simulink model "RCAMSimulation"  (R2025b)
settings: Solver=VariableStepAuto  StartTime=0.0  StopTime=TF  RelTol=1e-3
values from neighbouring files (symbols this model uses):
  u1max = 25*pi/180    (= 0.436332312999)    [Initialize_RCAM.m]
  u1min = -25*pi/180    (= -0.436332312999)    [Initialize_RCAM.m]
  u2max = 10*pi/180    (= 0.174532925199)    [Initialize_RCAM.m]
  u2min = -25*pi/180    (= -0.436332312999)    [Initialize_RCAM.m]
  u3max = 30*pi/180    (= 0.523598775598)    [Initialize_RCAM.m]
  u3min = -30*pi/180    (= -0.523598775598)    [Initialize_RCAM.m]
  u4max = 10*pi/180    (= 0.174532925199)    [Initialize_RCAM.m]
  u4min = 0    [Initialize_RCAM.m]
  u5max = 10*pi/180    (= 0.174532925199)    [Initialize_RCAM.m]
  u5min = 0.5*pi/180    (= 0.00872664625997)    [Initialize_RCAM.m]
  x0 = [85;0;0;0;0;0;0;0.1;0]    [Initialize_RCAM.m]
undefined symbols (not defined in the file or in its folder): RCAM_model
libraries: aerolibsim3d x2, sim3dlib x1
settings Model: Creator=andyf  LastModifiedBy=andyf

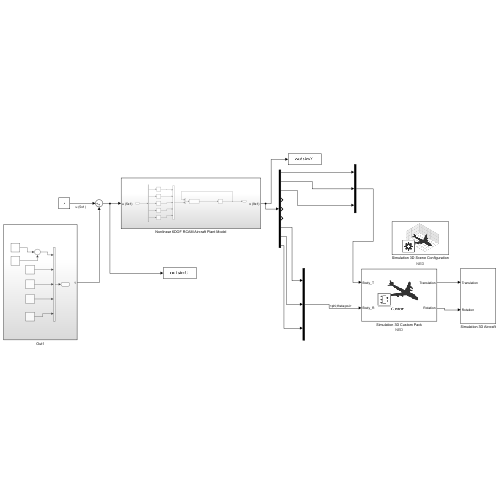
[thumbnail: Simulink's stored preview of the top-level diagram]
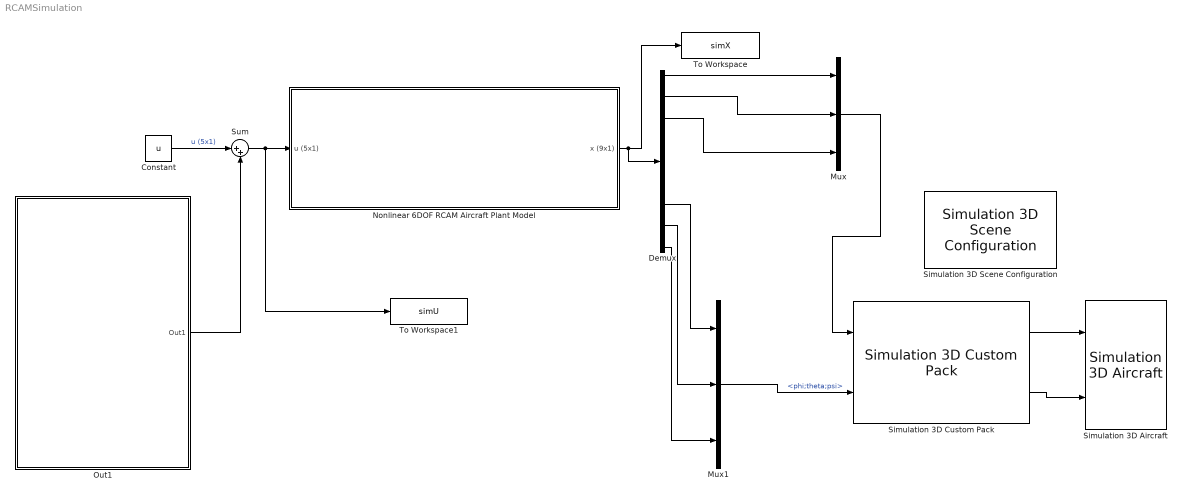
== system RCAMSimulation ==
  Constant : Constant  Value=u
  Demux : Demux  Outputs=9
  Mux : Mux  Inputs=3
  Mux1 : Mux  Inputs=3
  Nonlinear 6DOF RCAM Aircraft Plant Model : Subsystem
  Out1 : Subsystem
  Simulation 3D Aircraft : aerolibsim3d/Simulation 3D Aircraft  Priority=-1  Mesh=Custom  MeshPath=/MathWorksAerospaceContent/Vehicles/Aircraft/Custom/Mesh/SK_HL20.SK_HL20  MeshPathAT=/MathWorksAerospaceContent/Vehicles/Aircraft/AirTransport/Mesh/SK_AirTransport.SK_AirTransport  MeshPathGA=/MathWorksAerospaceContent/Vehicles/Aircraft/GeneralAviation/Mesh/SK_GeneralAviation.SK_GeneralAviation  AircraftColor=White  ActorName=SimulinkVehicle1  Translation=[-7000, 0, -3048; zeros( 56, 3 )]  Rotation=zeros( 57, 3 )  ScaleInputPort=Dialog  Scale=[1 1 1]  InitialScale=[1 1 1]  IsGHSensorEnabled=off  AreGHRaysVisible=off  IsOutputReshapeEnabled=off  GHRayLength=5000  GHBodyOffset=0.90  GHFrontTireRadius=0.21  GHLeftTireRadius=0.21  GHRightTireRadius=0.21  WoWSensorTolerance=0.05  LightsConfig=Automatic lights  LandingLightIntensity=300000  LandingLightConeAngle=15  CustomLeftLandingLightLocation=[0 0 0]  CustomLeftLandingLightOrientation=[0 0 0]  CustomRightLandingLightLocation=[0 0 0]  CustomRightLandingLightOrientation=[0 0 0]  TaxiLightIntensity=150000  TaxiLightConeAngle=36  CustomTaxiLightLocation=[0 0 0]  CustomTaxiLightOrientation=[0 0 0]  NavLightIntensity=500  PositionLightIntensity=500  StrobeLightIntensity=5000  WingtipStrobePeriod=1.5  WingtipStrobePulseWidth=6  TailStrobePeriod=1.5  TailStrobePulseWidth=6  BeaconLightIntensity=4000  BeaconPeriod=1.5  BeaconPulseWidth=10  SampleTime=-1  ActorType=SimulinkVehicle  ID=1  aMode=0  ActorTag=SimulinkVehicle1
  Simulation 3D Custom Pack : aerolibsim3d/Simulation 3D Custom Pack  Engine1_T=off  Engine1_R=off  Engine1_Prop_T=off  Engine1_Prop_R=off  Engine2_T=off  Engine2_R=off  Engine2_Prop_T=off  Engine2_Prop_R=off  Engine3_T=off  Engine3_R=off  Engine3_Prop_T=off  Engine3_Prop_R=off  Engine4_T=off  Engine4_R=off  Engine4_Prop_T=off  Engine4_Prop_R=off  Engine5_T=off  Engine5_R=off  Engine5_Prop_T=off  Engine5_Prop_R=off  Engine6_T=off  Engine6_R=off  Engine6_Prop_T=off  Engine6_Prop_R=off  Engine7_T=off  Engine7_R=off  Engine7_Prop_T=off  Engine7_Prop_R=off  Engine8_T=off  Engine8_R=off  Engine8_Prop_T=off  Engine8_Prop_R=off  Engine9_T=off  Engine9_R=off  Engine9_Prop_T=off  Engine9_Prop_R=off  Engine10_T=off  Engine10_R=off  Engine10_Prop_T=off  Engine10_Prop_R=off  Engine11_T=off  Engine11_R=off  Engine11_Prop_T=off  Engine11_Prop_R=off  Engine12_T=off  Engine12_R=off  Engine12_Prop_T=off  Engine12_Prop_R=off  Engine13_T=off  Engine13_R=off  Engine13_Prop_T=off  Engine13_Prop_R=off  Engine14_T=off  Engine14_R=off  Engine14_Prop_T=off  Engine14_Prop_R=off  Engine15_T=off  Engine15_R=off  Engine15_Prop_T=off  Engine15_Prop_R=off  Engine16_T=off  Engine16_R=off  Engine16_Prop_T=off  Engine16_Prop_R=off  Wing1_T=off  Wing1_R=off  Wing1_Left_Flap_T=off  Wing1_Left_Flap_R=off  Wing1_Right_Flap_T=off  Wing1_Right_Flap_R=off  Wing1_Left_Aileron_T=off  Wing1_Left_Aileron_R=off  Wing1_Right_Aileron_T=off  Wing1_Right_Aileron_R=off  Wing1_Left_Spoiler_T=off  Wing1_Left_Spoiler_R=off  Wing1_Right_Spoiler_T=off  Wing1_Right_Spoiler_R=off  Wing2_T=off  Wing2_R=off  Wing2_Left_Flap_T=off  Wing2_Left_Flap_R=off  Wing2_Right_Flap_T=off  Wing2_Right_Flap_R=off  Horizontal_Stab_T=off  Horizontal_Stab_R=off  Left_Elevator_T=off  Left_Elevator_R=off  Right_Elevator_T=off  Right_Elevator_R=off  Left_Rudder_T=off  Left_Rudder_R=off  Right_Rudder_T=off  Right_Rudder_R=off  Nose_Gear_T=off  Nose_Gear_R=off  Nose_Wheel_T=off  Nose_Wheel_R=off  Nose_Gear_Door_T=off  Nose_Gear_Door_R=off  Left_Gear_T=off  Left_Gear_R=off  Left_Wheel_T=off  Left_Wheel_R=off  Left_Gear_Door_T=off  Left_Gear_Door_R=off  Right_Gear_T=off  Right_Gear_R=off  Right_Wheel_T=off  Right_Wheel_R=off  Right_Gear_Door_T=off  Right_Gear_Door_R=off  EnableUETransform=on  GeoRadioButton=NED
      settings: AttributesFormatString=NED
  Simulation 3D Scene Configuration : sim3dlib/Simulation 3D Scene Configuration  Priority=0  ProjectFormat=Default Scenes  SceneDesc=Airport  ProjectName=C:\Program Files\MATLAB\R2025b\toolbox\shared\sim3d_projects\automotive_project_windows\UE\WindowsNoEditor\VehicleSimulation.exe  ScenePath=/Game/Maps/HwStrght  EnableOpenDRIVE=off  vehTagList={'Custom';'Scene Origin';'SimulinkVehicle1'}  vehTag=Custom  AttachedCameraRelativeTranslation=[0 0 0]  FreeCameraDefaultInitialTranslation=[-6, 0, 2]  AttachedCameraRelativeRotation=[0 0 0]  FreeCameraDefaultInitialRotation=[0, -15, 0]  ViewpointName=Custom  FreeCameraInitialTranslation=[0 0 0]  ViewpointTranslation=[0 0 0]  FreeCameraInitialRotation=[0 0 0]  ViewpointRotation=[0 0 0]  OpVisEn=off  Ts=1/60  EnableWindow=on  EnableRemoteAccess=off  EnableWeather=off  SunAzimuth=90  SunAltitude=40.0  EnableGeospatialSun=off  Latitude=0  Longitude=0  Date=2023-01-01  Time=10:30:00  GeoTimeZone=-5.0  SunDaylightSaving=off  wind=1  clouds=10  EnableVolumetricClouds=off  CloudCoverage=0  CloudAltitude=6  fog=0  rain=0  RaindropsEffect=off  SnowDensity=0  EnableGeospatial=off  TilesetSource=Earth terrain  UseTrueOrigin=off  OriginHeight=200  OriginLatitude=40.744652  OriginLongitude=-73.988864  MapStyle=Aerial  AdditionalAssetIDs=[]  UseAdvancedSunSky=off  SolarTime=11  TimeZone=-5  Day=21  Month=9  Year=2022  UseDaylightSavingTime=on  DSTStartDay=10  DSTStartMonth=3  DSTEndDay=3  DSTEndMonth=11  DSTSwitchHour=2  sensorTag=MainCamera1  sensorId=1  sensorName=MainCamera1  mountLoc=Origin  offsetFlag=off  tmountOffset=[0, 0, 0]  rmountOffset=[0, 0, 0]  HorizontalResolution=1280  VerticalResolution=720  HorizontalFOV=60  mountPoint=[0 0 0]  mountOrientation=[0 0 0]  aMode=0  ID=1  GeoTrigger=Inactive  ViewNameList={'Custom'}  ViewTranslationList={'[0 0 0]'}  ViewRotationList={'[0 0 0]'}
      settings: AttributesFormatString=NED  LibrarySourceBlock=aerolibsim3d/Simulation 3D Scene Configuration
  Sum : Sum  Inputs=|++
  To Workspace : ToWorkspace  VariableName=simX  SaveFormat=Timeseries  SampleTime=-1
  To Workspace1 : ToWorkspace  VariableName=simU  SaveFormat=Timeseries  SampleTime=-1
  wires:
  Nonlinear 6DOF RCAM Aircraft Plant Model/1(x (9x1)) -> Demux/1, To Workspace/1
  Constant/1 -> Sum/1  "u (5x1)"
  Out1/1(Out1) -> Sum/2
  Sum/1 -> To Workspace1/1, Nonlinear 6DOF RCAM Aircraft Plant Model/1(u (5x1))
  Mux1/1 -> Simulation 3D Custom Pack/2  "<phi;theta;psi>"
  Mux/1 -> Simulation 3D Custom Pack/1
  Demux/1 -> Mux/1
  Demux/2 -> Mux/2
  Demux/3 -> Mux/3
  Demux/7 -> Mux1/1
  Demux/8 -> Mux1/2
  Demux/9 -> Mux1/3
  Simulation 3D Custom Pack/1 -> Simulation 3D Aircraft/1
  Simulation 3D Custom Pack/2 -> Simulation 3D Aircraft/2

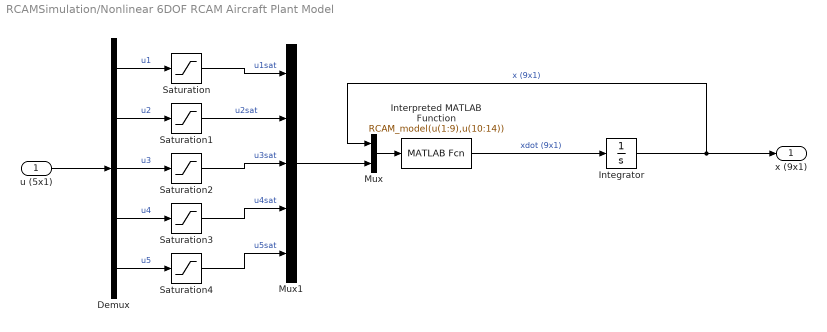
== system RCAMSimulation/Nonlinear 6DOF RCAM Aircraft Plant Model ==
  u (5x1) : Inport
  Demux : Demux  Outputs=5
  Integrator : Integrator  InitialCondition=x0
  Interpreted MATLAB Function : MATLABFcn  MATLABFcn=RCAM_model(u(1:9),u(10:14))
  Mux : Mux  Inputs=2
  Mux1 : Mux  Inputs=5
  Saturation : Saturate  UpperLimit=u1max  LowerLimit=u1min
  Saturation1 : Saturate  UpperLimit=u2max  LowerLimit=u2min
  Saturation2 : Saturate  UpperLimit=u3max  LowerLimit=u3min
  Saturation3 : Saturate  UpperLimit=u4max  LowerLimit=u4min
  Saturation4 : Saturate  UpperLimit=u5max  LowerLimit=u5min
  x (9x1) : Outport
  wires:
  Mux/1 -> Interpreted MATLAB Function/1
  Integrator/1 -> x (9x1)/1, Mux/1  "x (9x1)"
  Interpreted MATLAB Function/1 -> Integrator/1  "xdot (9x1)"
  u (5x1)/1 -> Demux/1
  Demux/1 -> Saturation/1  "u1"
  Saturation/1 -> Mux1/1  "u1sat"
  Demux/2 -> Saturation1/1  "u2"
  Demux/5 -> Saturation4/1  "u5"
  Demux/4 -> Saturation3/1  "u4"
  Demux/3 -> Saturation2/1  "u3"
  Saturation1/1 -> Mux1/2  "u2sat"
  Saturation2/1 -> Mux1/3  "u3sat"
  Saturation3/1 -> Mux1/4  "u4sat"
  Saturation4/1 -> Mux1/5  "u5sat"
  Mux1/1 -> Mux/2

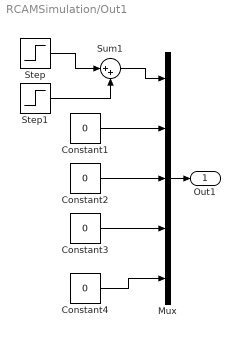
== system RCAMSimulation/Out1 ==
  Constant{1..4} (4 alike) : Constant  Value=0
  Mux : Mux  Inputs=5
  Step : Step  Time=30  After=5*pi/180  SampleTime=0
  Step1 : Step  Time=32  After=-5*pi/180  SampleTime=0
  Sum1 : Sum  Inputs=|++
  Out1 : Outport
  wires:
  Constant4/1 -> Mux/5
  Sum1/1 -> Mux/1
  Constant3/1 -> Mux/4
  Step1/1 -> Sum1/2
  Constant1/1 -> Mux/2
  Step/1 -> Sum1/1
  Constant2/1 -> Mux/3
  Mux/1 -> Out1/1
